simulink model "RadarSystemLevel"  (R2013a)
settings: Solver=FixedStepDiscrete  SolverMode=SingleTasking  StartTime=0.0  StopTime=4e-4  RelTol=1e-3
model workspace (MAT data in the model file):
  Ts = 1.6667e-07
  Ts1 = 1.6667e-07
  carrierFreq = 2100000000
  radar_system_bjt : rfckt.cascade (value not decoded)
undefined symbols (not defined in the file or in its folder): dfilt, magnitude
libraries: dspstat3 x6, dspmathops x5, rfports1 x2, rfladderfilters1 x1, rfmixers1 x1, rfamplifiers1 x1, rfmathmodels1 x1, commrflib2 x1, simulink x1, dsparch4 x1, dspsigops x1
settings Model: Creator=jbryan  LastModifiedBy=jbryan
settings DataIOCC: SaveOutput=off  SignalLogging=off  SaveTime=off
settings OptimizationCC: ExpressionDepthLimit=2147483647
settings DebuggingCC: AlgebraicLoopMsg=error  SingleTaskRateTransMsg=error

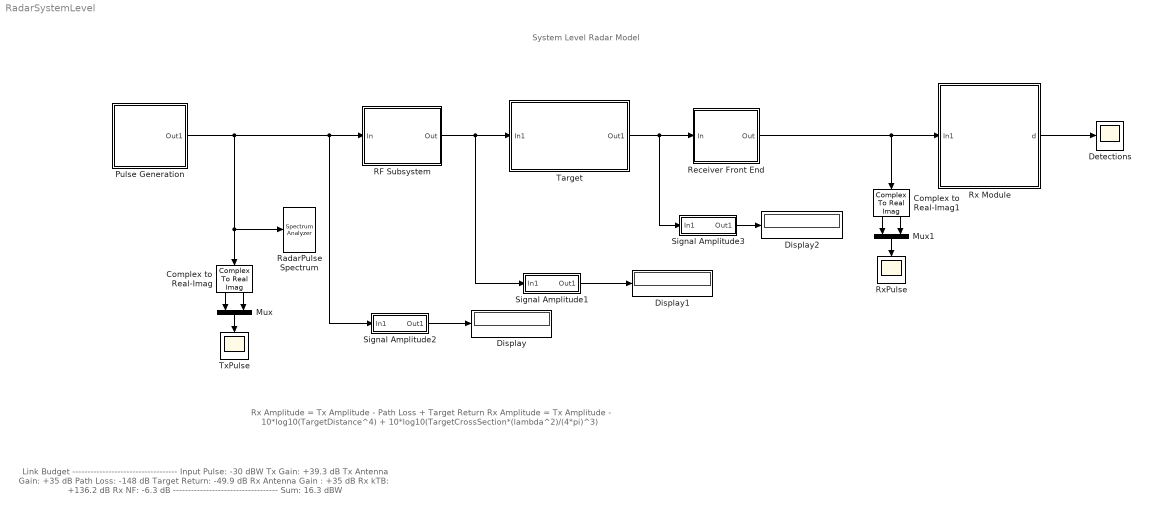
== system RadarSystemLevel ==
  note: Link Budget
      | -----------------------------------
      | Input Pulse:           -30 dBW
      | Tx Gain:                +39.3 dB
      | Tx Antenna Gain:     +35 dB
      | Path Loss:               -148 dB
      | Target Return:        -49.9 dB
      | Rx Antenna Gain :    +35 dB
      | Rx kTB:               +136.2 dB
      | Rx NF:                     -6.3 dB
      | -----------------------------------
      | Sum:                     16.3 dBW
  note: Rx Amplitude = Tx Amplitude - Path Loss + Target Return
      |
      | Rx Amplitude = Tx Amplitude - 10*log10(TargetDistance^4) + 10*log10(TargetCrossSection*(lambda^2)/(4*pi)^3)
  note: System Level Radar Model
  Complex to Real-Imag : ComplexToRealImag
  Complex to Real-Imag1 : ComplexToRealImag
  Detections : Scope
      settings: TimeRange=0.0004  YMin=0  YMax=1
  Display : Display
  Display1 : Display
  Display2 : Display
  Mux : Mux  Inputs=2
  Mux1 : Mux  Inputs=2
  Pulse Generation : Subsystem
      mask Display: image(imread('IC1.jpg'))
  RF Subsystem : Subsystem
      mask init:
      | sat = imread('satellite.jpg');
      | for ii=1:3, sat(:,:,ii) = fliplr(sat(:,:,ii)); end;
      mask Display: image(sat)
  RadarPulse Spectrum : SpectrumAnalyzer
      settings: CopyFcn=scopeextensions.ScopeBlock.callback(gcbh, 'onBlockCopy', gcbh);  DeleteFcn=scopeextensions.ScopeBlock.callback(gcbh, 'onBlockDelete');  PreSaveFcn=scopeextensions.ScopeBlock.callback(gcbh, 'onModelSave');  NameChangeFcn=scopeextensions.ScopeBlock.callback(gcbh, 'onBlockRename');  CloseFcn=scopeextensions.ScopeBlock.callback(gcbh, 'onBlockClose');  PreDeleteFcn=scopeextensions.ScopeBlock.callback(gcbh, 'onBlockPreDelete');
  Receiver Front End : Subsystem
      mask Display: image(imread('cobradane.jpg'))
  Rx Module : Subsystem
      mask Display: image(imread('RxBoard1.jpg'))
  RxPulse : Scope
      settings: TimeRange=0.0004  YMin=-4e-05  YMax=5e-05  SaveName=ScopeData2
  Signal Amplitude1 : Subsystem
  Signal Amplitude2 : Subsystem
  Signal Amplitude3 : Subsystem
  Target : Subsystem  mask(Target){DistanceStart=5000, Speed=0, RCS=1, cf=carrierFreq}
      mask prompts: DistanceStart "Starting distance (m)"; Speed "Velocity (m/s)"; RCS "Radar cross section (m^2)"; cf "Carrier Frequency (Hz)"
      mask init:
      | lambda=3e8/cf; % Speed/Frequency;
      | Doppler=Speed/lambda; % Doppler shift Vehicle speed/Wavelength
      | ufo = imread('ufo.jpg','jpeg');
      mask Display: image(ufo);
  TxPulse : Scope
      settings: TimeRange=0.0004  YMin=0  YMax=0.035
  wires:
  Rx Module/1(d) -> Detections/1
  RF Subsystem/1(Out) -> Signal Amplitude1/1(In1), Target/1(In1)
  Signal Amplitude2/1(Out1) -> Display/1
  Target/1(Out1) -> Signal Amplitude3/1(In1), Receiver Front End/1(In)
  Signal Amplitude1/1(Out1) -> Display1/1
  Signal Amplitude3/1(Out1) -> Display2/1
  Pulse Generation/1(Out1) -> Complex to Real-Imag/1, RadarPulse Spectrum/1, Signal Amplitude2/1(In1), RF Subsystem/1(In)
  Complex to Real-Imag/1 -> Mux/1
  Complex to Real-Imag/2 -> Mux/2
  Mux/1 -> TxPulse/1
  Receiver Front End/1(Out) -> Complex to Real-Imag1/1, Rx Module/1(In1)
  Complex to Real-Imag1/1 -> Mux1/1
  Complex to Real-Imag1/2 -> Mux1/2
  Mux1/1 -> RxPulse/1

== system RadarSystemLevel/Pulse Generation ==
  MATLAB Function : MATLAB Function  TreatAsAtomicUnit=on
  "Normalize to 1mW @ 1 Ohms " : Gain  Gain=sqrt(.001)
  Out1 : Outport
  wires:
  MATLAB Function/1(y) -> "Normalize to 1mW @ 1 Ohms "/1
  "Normalize to 1mW @ 1 Ohms "/1 -> Out1/1

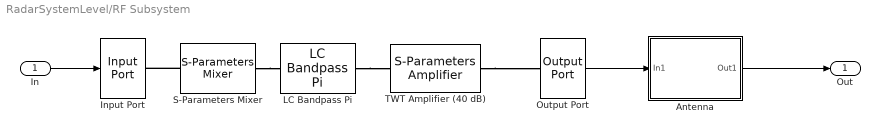
== system RadarSystemLevel/RF Subsystem ==
  In : Inport
  Antenna : Subsystem
  Input Port : rfports1/Input Port  Description=source block  TreatSimulinkInputSignalAs=Incident power wave  MaxLength=128  FracBW=0  ModelDelay=0  Fc=carrierFreq  Ts=Ts  Zs=50  RFhasDSP=Columns as channels (frame based)  NoiseFlag=off  seed=67987  GoToTag=ACDAIAASQCZHIWAEGFXIUVU
  LC Bandpass Pi : rfladderfilters1/LC Bandpass Pi  LConnTagsString=__newl0  RConnTagsString=__newr0  L="[1.4446e-9  4.3949e-8  1.4446e-9]*.32"  C="[3.5785e-11  1.1762e-12  3.5785e-11]*.32"  PlotFreq=User-specified  SourceFreq=User-specified  Freq=[1000e6:4e6:3000e6]  AllPlotType=X-Y plane  AppliedNetworkData=S21  AppliedComplexFormat=Magnitude (decibels)  AppliedNetworkData2=""  AppliedXParameter=Freq  AppliedXFormat=Hz  YOption=Linear  XOption=Linear  PlotZ0=50  DisplayData=off  PlotFreqNoSim=User-specified  NetworkData=S21  SmithData=S11  PolarData=S11  ComplexFormat=Magnitude (decibels)  DBFormat=Magnitude (decibels)  NoneFormat=None
  Output Port : rfports1/Output Port  Zl=50  Flag=1  num_Models=0  GoToTag=ACDAIAASQCZHIWAEGFXIUVU  PlotFreq=User-specified  SourceFreq=Derived from Input Port parameters  Freq=1e9:1e8:3e9  AllPlotType=X-Y plane  AppliedNetworkData=S21  AppliedComplexFormat=Magnitude (decibels)  AppliedNetworkData2=NF  AppliedComplexFormat2=Magnitude (decibels)  AppliedXParameter=Freq  AppliedXFormat=Hz  YOption=Linear  XOption=Linear  PlotZ0=50  DisplayData=off  NoBudgetPlot=Composite data  NetworkData=S11  SmithData=S11  PolarData=S11  ComplexFormat=Magnitude (decibels)  DBFormat=Magnitude (decibels)  DBMFormat=dBm  NoneFormat=None
  S-Parameters Mixer : rfmixers1/S-Parameters Mixer  LConnTagsString=__newl0  RConnTagsString=__newr0  NetParamData=[0 0;1 0]  NetParamFreq=carrierFreq  Z0=50  InterpMethod=Linear  MixerType=Upconverter  FLO=0  IP3Type=OIP3  IIP3=inf  OIP3=inf  P1dB=inf  PSat=inf  GCSat=0  NonlinearDataFreq=2.0e9  NoiseDefinedBy=Noise figure  NF=0  FMIN=0  GammaOpt=1  RN=1  NFactor=1  NTemp=0  NoiseDataFreq=2.0e9  FreqOffset=[0.1 1 10 100]*1e3  PhaseNoiseLevel=[-70 -120 -140 -150]  PlotFreq=Same as the Frequency parameter  SourceFreq=Same as the s-parameters frequency  Freq=[1e9:1e8:2.9e9]  SourcePin=Extracted from data source  Pin=0  AllPlotType=X-Y plane  AppliedNetworkData=S11  AppliedComplexFormat=Magnitude (decibels)  AppliedNetworkData2=""  AppliedComplexFormat2=""  AppliedXParameter=Freq  AppliedXFormat=Auto  YOption=Linear  XOption=Linear  PlotZ0=50  PlotFreqNoSim=0  DisplayData=0  NetworkData=0  SmithData=0  PolarData=0  ComplexFormat=0  DBFormat=0  NoneFormat=0  DBcFormat=0
  TWT Amplifier (40 dB) : rfamplifiers1/S-Parameters Amplifier  LConnTagsString=__newl0  RConnTagsString=__newr0  NetParamData=[0,0;sqrt(10000),0]  NetParamFreq=carrierFreq  Z0=50  InterpMethod=Linear  IP3Type=OIP3  IIP3=50  OIP3=50  P1dB=inf  PSat=inf  GCSat=0  NonlinearDataFreq=2.0e9  NoiseDefinedBy=Noise figure  NF=8  FMIN=0  GammaOpt=1  RN=1  NFactor=1  NTemp=0  NoiseDataFreq=2.0e9  PlotFreq=Derived from Input Port parameters  SourceFreq=Same as the s-parameters frequency  Freq=[1.9e9:1.0e8:2.2e9]  SourcePin=Extracted from data source  Pin=0  AllPlotType=X-Y plane  AppliedNetworkData=S11  AppliedComplexFormat=Magnitude (decibels)  AppliedNetworkData2=""  AppliedComplexFormat2=""  AppliedXParameter=Freq  AppliedXFormat=Auto  YOption=Linear  XOption=Linear  PlotZ0=50  PlotFreqNoSim=0  DisplayData=0  NetworkData=0  SmithData=0  PolarData=0  ComplexFormat=0  DBFormat=0  NoneFormat=0
  Out : Outport
  wires:
  Antenna/1(Out1) -> Out/1
  Output Port/1 -> Antenna/1(In1)
  In/1 -> Input Port/1
  connections:
  S-Parameters Mixer/RConn1 -- LC Bandpass Pi/LConn1
  S-Parameters Mixer/LConn1 -- Input Port/RConn1
  TWT Amplifier (40 dB)/RConn1 -- Output Port/LConn1
  LC Bandpass Pi/RConn1 -- TWT Amplifier (40 dB)/LConn1

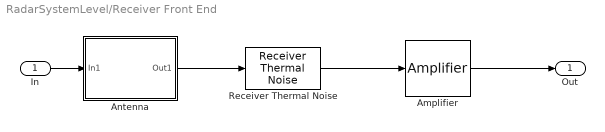
== system RadarSystemLevel/Receiver Front End ==
  In : Inport
  Amplifier : rfmathmodels1/Amplifier  model_select=Linear  linGaindB=30  GindB=0  iip3=30  am2pm=10  PwrAMPMStart=10  PwrAMPMEnd=inf  amam=[2.1587 1.1517]  ampm=[4.0033 9.1040]  x=[8.1081 1.5413 6.5202 -0.0718]  y=[4.6645 2.0965 10.88 -0.003]  p=0.5  GoutdB=0  vsat=1  method_select=Noise figure  ntemp=290  nfigure=6.3  nfactor=6.3  seed=67987
  Antenna : Subsystem
  Receiver Thermal Noise : commrflib2/Receiver Thermal Noise  method=Noise temperature  ntemp=290  nfigure=3.01  nfactor=2  seed=67987
  Out : Outport
  wires:
  In/1 -> Antenna/1(In1)
  Antenna/1(Out1) -> Receiver Thermal Noise/1
  Receiver Thermal Noise/1 -> Amplifier/1
  Amplifier/1 -> Out/1

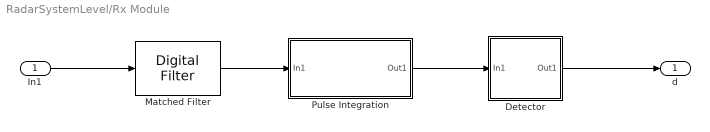
== system RadarSystemLevel/Rx Module ==
  In1 : Inport
  Detector : Subsystem
  Matched Filter : dsparch4/Digital Filter  TypePopup=FIR (all zeros)  IIRFiltStruct=Direct form II transposed  AllPoleFiltStruct=Direct form  FIRFiltStruct=Direct form  CoeffSource=Specify via dialog  NumCoeffs=[1 1]  DenCoeffs=[1 0.1]  BiQuadCoeffs=[1 0.3 0.4 1 0.1 0.2]  LatticeCoeffs=[0.2 0.4]  denIgnore=on  FiltPerSampPopup=One filter per frame  IC=0  ICnum=0  ICden=0  roundingMode=Floor  overflowMode=off  ScaleValues=1  scaleValueFracLength=14  stageInFracLength=15  stageOutFracLength=15  FilterSource=Specify via dialog  dfiltObjectName=dfilt.dffir([1 2 1])  InputProcessing=Columns as channels (frame based)
  Pulse Integration : Subsystem  mask(Noncoherent pulse integration){pulseLen=200, N=10}
      mask prompts: pulseLen "Pulse length (samples)"; N "Number of pulses"
  d : Outport
  wires:
  In1/1 -> Matched Filter/1
  Matched Filter/1 -> Pulse Integration/1(In1)
  Detector/1(Out1) -> d/1
  Pulse Integration/1(Out1) -> Detector/1(In1)

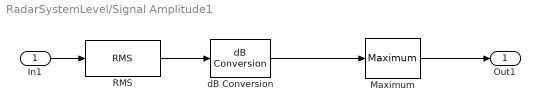
== system RadarSystemLevel/Signal Amplitude1 ==
  In1 : Inport
  Maximum : dspstat3/Maximum  fcn=Running  reset=None  indexBase=One  operateOver=Each column  Dimension=1  colComp=on  operation=maximum  roiEnable=off  roiType=Rectangles  roiPortion=Entire ROI  roiOutput=Individual statistics for each ROI  roiFlag=off  accumDataTypeStr=Inherit: Same as product output  accumLastDataTypeStr=Inherit: Same as product output  roundingMode=Floor  overflowMode=off
  RMS : dspstat3/RMS  run=off  reset_popup=None  InputProcessing=Columns as channels (frame based)  directionMode=Each column  dimension=1  treatSBRowAsCol=on
  dB Conversion : dspmathops/dB Conversion  dBtype=dB  intype=Amplitude  R=1  fuzz=off
  Out1 : Outport
  wires:
  dB Conversion/1 -> Maximum/1
  RMS/1 -> dB Conversion/1
  In1/1 -> RMS/1
  Maximum/1 -> Out1/1

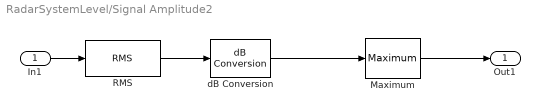
== system RadarSystemLevel/Signal Amplitude2 ==
  In1 : Inport
  Maximum : dspstat3/Maximum  fcn=Running  reset=None  indexBase=One  operateOver=Each column  Dimension=1  colComp=on  operation=maximum  roiEnable=off  roiType=Rectangles  roiPortion=Entire ROI  roiOutput=Individual statistics for each ROI  roiFlag=off  accumDataTypeStr=Inherit: Same as product output  accumLastDataTypeStr=Inherit: Same as product output  roundingMode=Floor  overflowMode=off
  RMS : dspstat3/RMS  run=off  reset_popup=None  InputProcessing=Columns as channels (frame based)  directionMode=Each column  dimension=1  treatSBRowAsCol=on
  dB Conversion : dspmathops/dB Conversion  dBtype=dB  intype=Amplitude  R=1  fuzz=off
  Out1 : Outport
  wires:
  Maximum/1 -> Out1/1
  In1/1 -> RMS/1
  RMS/1 -> dB Conversion/1
  dB Conversion/1 -> Maximum/1

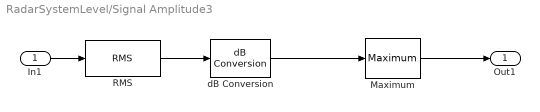
== system RadarSystemLevel/Signal Amplitude3 ==
  In1 : Inport
  Maximum : dspstat3/Maximum  fcn=Running  reset=None  indexBase=One  operateOver=Each column  Dimension=1  colComp=on  operation=maximum  roiEnable=off  roiType=Rectangles  roiPortion=Entire ROI  roiOutput=Individual statistics for each ROI  roiFlag=off  accumDataTypeStr=Inherit: Same as product output  accumLastDataTypeStr=Inherit: Same as product output  roundingMode=Floor  overflowMode=off
  RMS : dspstat3/RMS  run=off  reset_popup=None  InputProcessing=Columns as channels (frame based)  directionMode=Each column  dimension=1  treatSBRowAsCol=on
  dB Conversion : dspmathops/dB Conversion  dBtype=dB  intype=Amplitude  R=1  fuzz=off
  Out1 : Outport
  wires:
  Maximum/1 -> Out1/1
  In1/1 -> RMS/1
  RMS/1 -> dB Conversion/1
  dB Conversion/1 -> Maximum/1

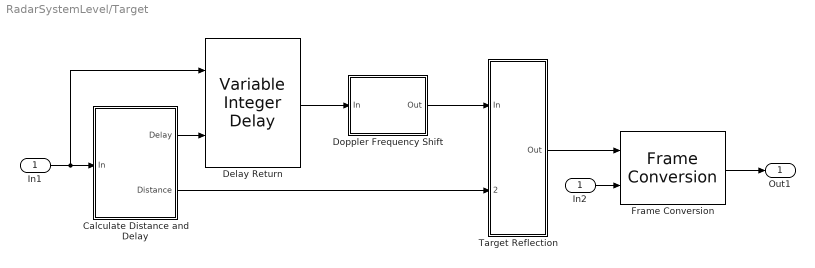
== system RadarSystemLevel/Target ==
  In1 : Inport
  Calculate Distance and Delay : Subsystem
  Delay Return : dspsigops/Variable Integer Delay  dmax=10000  InputProcessing=Columns as channels (frame based)  ic=0  noDFT=off
  Doppler Frequency Shift : Subsystem
  Frame Conversion : FrameConversion  InheritSamplingMode=on
  In2 : InportShadow
  Target Reflection : Subsystem
  Out1 : Outport
  wires:
  In2/1 -> Frame Conversion/2
  Frame Conversion/1 -> Out1/1
  Target Reflection/1(Out) -> Frame Conversion/1
  Doppler Frequency Shift/1(Out) -> Target Reflection/1(In)
  In1/1 -> Delay Return/1, Calculate Distance and Delay/1(In)
  Calculate Distance and Delay/2(Distance) -> Target Reflection/2(Distance)
  Delay Return/1 -> Doppler Frequency Shift/1(In)
  Calculate Distance and Delay/1(Delay) -> Delay Return/2

== system RadarSystemLevel/RF Subsystem/Antenna ==
  In1 : Inport
  dB Gain : dspmathops/dB Gain  dB=35  intype=Amplitude
  Out1 : Outport
  wires:
  dB Gain/1 -> Out1/1
  In1/1 -> dB Gain/1

== system RadarSystemLevel/Receiver Front End/Antenna ==
  In1 : Inport
  dB Gain : dspmathops/dB Gain  dB=35  intype=Amplitude
  Out1 : Outport
  wires:
  dB Gain/1 -> Out1/1
  In1/1 -> dB Gain/1

== system RadarSystemLevel/Rx Module/Detector ==
  In1 : Inport
  Threshold : simulink/Logic and Bit Operations/Compare To Constant  relop=>  const=1e-4  OutDataTypeStr=boolean
  Out1 : Outport
  wires:
  In1/1 -> Threshold/1
  Threshold/1 -> Out1/1

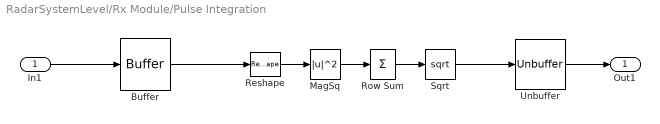
== system RadarSystemLevel/Rx Module/Pulse Integration ==
  In1 : Inport
  Buffer : Buffer  N=pulseLen*N  V=pulseLen*(N-1)  TreatMby1Signals=One channel
  MagSq : Math  Operator=magnitude^2  SaturateOnIntegerOverflow=on
  Reshape : Reshape  OutputDimensionality=Customize  OutputDimensions=[pulseLen,N]
  Row Sum : Sum  Inputs=+  CollapseMode=Specified dimension  CollapseDim=2
  Sqrt : Sqrt  SaturateOnIntegerOverflow=on
  Unbuffer : Unbuffer  SampleBasedProcessing=Same as frame based
  Out1 : Outport
  wires:
  Sqrt/1 -> Unbuffer/1
  Unbuffer/1 -> Out1/1
  Buffer/1 -> Reshape/1
  Row Sum/1 -> Sqrt/1
  In1/1 -> Buffer/1
  Reshape/1 -> MagSq/1
  MagSq/1 -> Row Sum/1

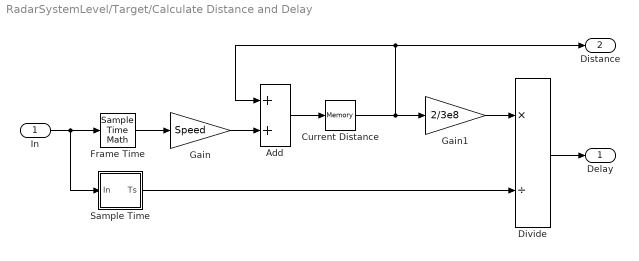
== system RadarSystemLevel/Target/Calculate Distance and Delay ==
  In : Inport
  Add : Sum
  Current Distance : Memory  X0=DistanceStart  InheritSampleTime=on
  Divide : Product  Inputs=*/
  Frame Time : SampleTimeMath  TsampMathOp=Ts Only
  Gain : Gain  Gain=Speed  SaturateOnIntegerOverflow=on  OutDataTypeStr=Inherit: Same as input  ParamDataTypeStr=Inherit: Same as input
  Gain1 : Gain  Gain=2/3e8
  Sample Time : Subsystem
  Delay : Outport
  Distance : Outport  Port=2
  wires:
  Sample Time/1(Ts) -> Divide/2
  Gain/1 -> Add/2
  Current Distance/1 -> Distance/1, Add/1, Gain1/1
  Add/1 -> Current Distance/1
  Gain1/1 -> Divide/1
  Frame Time/1 -> Gain/1
  In/1 -> Sample Time/1(In), Frame Time/1
  Divide/1 -> Delay/1

== system RadarSystemLevel/Target/Doppler Frequency Shift ==
  In : Inport
  Doppler Frequency Shift : MATLAB Function  TreatAsAtomicUnit=on
  Sample Time : Subsystem
  Out : Outport
  wires:
  Doppler Frequency Shift/1(y) -> Out/1
  Sample Time/1(Ts) -> Doppler Frequency Shift/2(Ts)
  In/1 -> Doppler Frequency Shift/1(u), Sample Time/1(In)

== system RadarSystemLevel/Target/Target Reflection ==
  In : Inport
  Distance : Inport  Port=2
  Target Reflection : MATLAB Function  TreatAsAtomicUnit=on
  Out : Outport
  wires:
  Distance/1 -> Target Reflection/2(Distance)
  Target Reflection/1(y) -> Out/1
  In/1 -> Target Reflection/1(u)

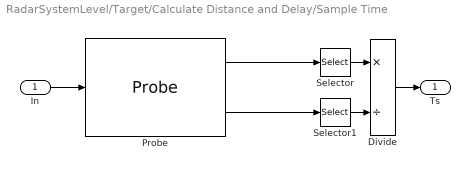
== system RadarSystemLevel/Target/Calculate Distance and Delay/Sample Time ==
  In : Inport
  Divide : Product  Inputs=*/
  Probe : Probe  ProbeWidth=off  ProbeComplexSignal=off  ProbeSignalDimensions=on
  Selector : Selector  InputPortWidth=2  IndexOptions=Index vector (dialog)  Indices=1  OutputSizes=1
  Selector1 : Selector  InputPortWidth=2  IndexOptions=Index vector (dialog)  Indices=1  OutputSizes=1
  Ts : Outport
  wires:
  Divide/1 -> Ts/1
  In/1 -> Probe/1
  Selector1/1 -> Divide/2
  Selector/1 -> Divide/1
  Probe/2 -> Selector1/1
  Probe/1 -> Selector/1

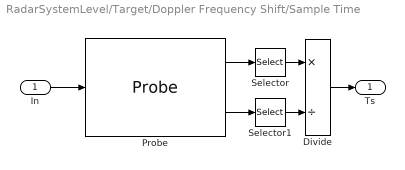
== system RadarSystemLevel/Target/Doppler Frequency Shift/Sample Time ==
  In : Inport
  Divide : Product  Inputs=*/
  Probe : Probe  ProbeWidth=off  ProbeComplexSignal=off  ProbeSignalDimensions=on
  Selector : Selector  InputPortWidth=2  IndexOptions=Index vector (dialog)  Indices=1  OutputSizes=1
  Selector1 : Selector  InputPortWidth=2  IndexOptions=Index vector (dialog)  Indices=1  OutputSizes=1
  Ts : Outport
  wires:
  Probe/1 -> Selector/1
  Probe/2 -> Selector1/1
  Selector/1 -> Divide/1
  Selector1/1 -> Divide/2
  In/1 -> Probe/1
  Divide/1 -> Ts/1

== matlab function RadarSystemLevel/Target/Doppler Frequency Shift/Doppler Frequency Shift ==
  data: u input; y output; Doppler parameter; Ts input
function y = fcn(u,Doppler,Ts)
% Doppler frequency shift

y = exp(1j*2*pi*Doppler*Ts*(1:length(u))).'.*u;

== matlab function RadarSystemLevel/Pulse Generation/MATLAB Function ==
  settings: updateMethod=DISCRETE  sampleTime=Ts
  data: y output
function y = fcn()
%#codegen

y = waveform_rect();

== matlab function RadarSystemLevel/Target/Target Reflection/Target Reflection ==
  data: u input; y output; Distance input; RCS parameter; lambda parameter
function y = fcn(u,Distance,RCS,lambda)
% Target Reflection 

y = u.*sqrt(1./Distance.^4).*sqrt((lambda^2*RCS/(4*pi)^3));
%y = u.*(1./Distance.^4).*((lambda^2*RCS/(4*pi)^3));
